simulink model "RoboBoatVU_2014_F"  (R2014a)
settings: Solver=FixedStepDiscrete  StartTime=0.0  StopTime=inf  FixedStep=.1  RelTol=1e-3
undefined symbols (not defined in the file): Com1, Com2, Com3, Com4, DiscIntNeverNeededParam, RGB24, standard
libraries: visiontextngfix x74, simulink x56, xpcseriallib x15, dspmtrx3 x14, slrtlib x3, speedgoatlib_IO102 x3, visionstatistics x2, dspstat3 x2, dspindex x2, xpcvideousblib x2, xpcvideoutillib x2, speedgoatlib x1
(part 7 of 7)

== system RoboBoatVU_2014_F/Main FSM/Start Speed Gate/Start Speed Gate Detection/Green Detection/Image Reduction ==
  HSV : Inport
  Cut Out Sky : dspmtrx3/Submatrix  RowSpan=Range of rows  RowStartMode=First  RowStartIndex=1  RowEndMode=Index  RowEndIndex=280  ColSpan=Range of columns  ColStartMode=First  ColStartIndex=1  ColEndMode=Last  ColEndIndex=1
  Cut Out Sky1 : dspmtrx3/Submatrix  RowSpan=Range of rows  RowStartMode=First  RowStartIndex=1  RowEndMode=Index  RowEndIndex=280  ColSpan=Range of columns  ColStartMode=First  ColStartIndex=1  ColEndMode=Last  ColEndIndex=1
  H : Selector  NumberOfDimensions=3  InputPortWidth=3  IndexOptions=Select all,Select all,Index vector (dialog)  Indices=[1 3],1,1  OutputSizes=1,1,1
  Logical Operator : Logic  AllPortsSameDT=off  OutDataTypeStr=boolean
  Logical Operator1 : Logic  AllPortsSameDT=off  OutDataTypeStr=boolean
  Logical Operator2 : Logic  AllPortsSameDT=off  OutDataTypeStr=boolean
  Upper limit : simulink/Logic and Bit Operations/Compare To Constant  relop=<=  const=110  OutDataTypeStr=boolean
  Upper limit1 : simulink/Logic and Bit Operations/Compare To Constant  relop=>=  const=90  OutDataTypeStr=boolean
  Upper limit2 : simulink/Logic and Bit Operations/Compare To Constant  relop=>=  const=60  OutDataTypeStr=boolean
  Upper limit3 : simulink/Logic and Bit Operations/Compare To Constant  relop=<=  const=160  OutDataTypeStr=boolean
  V : Selector  NumberOfDimensions=3  InputPortWidth=3  IndexOptions=Select all,Select all,Index vector (dialog)  Indices=[1 3],1,3  OutputSizes=1,1,1
  Green BW : Outport
  wires:
  H/1 -> Cut Out Sky/1
  HSV/1 -> V/1, H/1
  Cut Out Sky/1 -> Upper limit1/1, Upper limit/1
  Upper limit1/1 -> Logical Operator/2
  Upper limit/1 -> Logical Operator/1
  V/1 -> Cut Out Sky1/1
  Cut Out Sky1/1 -> Upper limit3/1, Upper limit2/1
  Logical Operator/1 -> Logical Operator1/1
  Logical Operator1/1 -> Green BW/1
  Upper limit2/1 -> Logical Operator2/1
  Upper limit3/1 -> Logical Operator2/2
  Logical Operator2/1 -> Logical Operator1/2

== system RoboBoatVU_2014_F/Main FSM/Start Speed Gate/Start Speed Gate Detection/Red Detection/Exclusions ==
  Area In : Inport
  Centroid In : Inport  Port=2
  BBox In : Inport  Port=3
  Extent In : Inport  Port=4
  Closest Blob : Subsystem
  Data Type Conversion : DataTypeConversion  OutDataTypeStr=double
  Extent Exclusion : Subsystem
  Height to Width Exclusion : Subsystem
  Logical Operator : Logic  AllPortsSameDT=off  OutDataTypeStr=boolean
  Variable Selector : dspindex/Variable Selector  NumInputs=3  rowsOrCols=Rows  IdxMode=Variable  Elements=[1 3]  ZerOneIdxMode=One-based  errmode=Clip Index  FillMode=on  FillValues=-1
  Centroid Out : Outport
  BBox Out : Outport  Port=2
  wires:
  Extent In/1 -> Extent Exclusion/1(Extent)
  BBox In/1 -> Data Type Conversion/1
  Height to Width Exclusion/1(Idx) -> Logical Operator/1
  Extent Exclusion/1(Idx) -> Logical Operator/2
  Logical Operator/1 -> Variable Selector/4
  Centroid In/1 -> Variable Selector/2
  Variable Selector/2 -> Closest Blob/2(Centroid In)
  Variable Selector/3 -> Closest Blob/3(BBox In)
  Closest Blob/1(Centroid Out) -> Centroid Out/1
  Closest Blob/2(BBox Out) -> BBox Out/1
  Data Type Conversion/1 -> Variable Selector/3, Height to Width Exclusion/1(BBox)
  Area In/1 -> Variable Selector/1
  Variable Selector/1 -> Closest Blob/1(Area In)

== system RoboBoatVU_2014_F/Main FSM/Start Speed Gate/Start Speed Gate Detection/Red Detection/Image Reduction ==
  HSV : Inport
  Cut Out Sky : dspmtrx3/Submatrix  RowSpan=Range of rows  RowStartMode=First  RowStartIndex=1  RowEndMode=Index  RowEndIndex=280  ColSpan=Range of columns  ColStartMode=First  ColStartIndex=1  ColEndMode=Last  ColEndIndex=1
  Cut Out Sky1 : dspmtrx3/Submatrix  RowSpan=Range of rows  RowStartMode=First  RowStartIndex=1  RowEndMode=Index  RowEndIndex=280  ColSpan=Range of columns  ColStartMode=First  ColStartIndex=1  ColEndMode=Last  ColEndIndex=1
  H : Selector  NumberOfDimensions=3  InputPortWidth=3  IndexOptions=Select all,Select all,Index vector (dialog)  Indices=[1 3],1,1  OutputSizes=1,1,1
  H Range 1 : simulink/Logic and Bit Operations/Compare To Constant  relop=<=  const=5  OutDataTypeStr=boolean
  H Range 2 : simulink/Logic and Bit Operations/Compare To Constant  relop=>=  const=0  OutDataTypeStr=boolean
  H Range 3 : simulink/Logic and Bit Operations/Compare To Constant  relop=<=  const=255  OutDataTypeStr=boolean
  H Range 4 : simulink/Logic and Bit Operations/Compare To Constant  relop=>=  const=220  OutDataTypeStr=boolean
  Logical Operator{,1,3..4} (4 alike) : Logic  AllPortsSameDT=off  OutDataTypeStr=boolean
  Logical Operator2 : Logic  Operator=OR  AllPortsSameDT=off  OutDataTypeStr=boolean
  V : Selector  NumberOfDimensions=3  InputPortWidth=3  IndexOptions=Select all,Select all,Index vector (dialog)  Indices=[1 3],1,3  OutputSizes=1,1,1
  V Range : simulink/Logic and Bit Operations/Compare To Constant  relop=>=  const=60  OutDataTypeStr=boolean
  V Range1 : simulink/Logic and Bit Operations/Compare To Constant  relop=<=  const=200  OutDataTypeStr=boolean
  Red BW : Outport
  wires:
  HSV/1 -> H/1, V/1
  H/1 -> Cut Out Sky/1
  Cut Out Sky/1 -> H Range 4/1, H Range 3/1, H Range 2/1, H Range 1/1
  V/1 -> Cut Out Sky1/1
  H Range 1/1 -> Logical Operator/1
  H Range 2/1 -> Logical Operator/2
  H Range 3/1 -> Logical Operator1/1
  H Range 4/1 -> Logical Operator1/2
  Logical Operator/1 -> Logical Operator2/1
  Logical Operator1/1 -> Logical Operator2/2
  Cut Out Sky1/1 -> V Range1/1, V Range/1
  Logical Operator2/1 -> Logical Operator3/1
  Logical Operator3/1 -> Red BW/1
  V Range/1 -> Logical Operator4/1
  V Range1/1 -> Logical Operator4/2
  Logical Operator4/1 -> Logical Operator3/2

== system RoboBoatVU_2014_F/Sinks/actuators/analog output/Subsystem/Heading Controller ==
  Heading Desired : Inport
  Compass Heading : Inport  Port=2
  Gain : Gain  Gain=-0.05
  MATLAB Function : MATLAB Function  TreatAsAtomicUnit=on
  Saturation : Saturate  UpperLimit=5  LowerLimit=0
  Sum : Sum  Inputs=++|
  Voltage Nuetral : Constant  Value=2.5
  Steering : Outport
  wires:
  Compass Heading/1 -> MATLAB Function/2(CompassHeading)
  Heading Desired/1 -> MATLAB Function/1(HeadingDesired)
  MATLAB Function/1(steering) -> Gain/1
  Gain/1 -> Sum/2
  Voltage Nuetral/1 -> Sum/1
  Sum/1 -> Saturation/1
  Saturation/1 -> Steering/1

== system RoboBoatVU_2014_F/Sinks/actuators/analog output/Subsystem/Propulsion Controller ==
  RPM : Inport
  Saturation : Saturate  UpperLimit=5  LowerLimit=0
  Sum : Sum  Inputs=++|
  Voltage Neutral : Constant  Value=2.5
  Volts / RPM : Gain  Gain=2.5/6000
  Propulsion : Outport
  wires:
  RPM/1 -> Volts / RPM/1
  Volts / RPM/1 -> Sum/2
  Voltage Neutral/1 -> Sum/1
  Sum/1 -> Saturation/1
  Saturation/1 -> Propulsion/1

== system RoboBoatVU_2014_F/Main FSM/Obstacle Navigation1/Obstacle Navigation/GPS: Bee Line/Approach/Output Heirarchy ==
  Nav Finished : Inport
  Desired Heading : Inport  Port=2
  Sensors : Inport  Port=3
  Annotated Image : Inport  Port=4
  Bus Creator : BusCreator  Inputs=3
  Bus Creator1 : BusCreator  Inputs=2
  Bus Creator2 : BusCreator  Inputs=3
  Bus Creator3 : BusCreator  Inputs=2
  Bus Creator4 : BusCreator  Inputs=2
  Due Sample Start : Constant  Value=0
  RPM Desired : Constant  Value=2000
  Ready to Read : Constant  Value=0
  Uno Power : Constant  Value=0
  Outputs : Outport
  wires:
  RPM Desired/1 -> Bus Creator/1  "RPM"
  Bus Creator/1 -> Bus Creator1/1  "Control Signals"
  Bus Creator2/1 -> Bus Creator/3  "Arduino Signals"
  Uno Power/1 -> Bus Creator2/2  "Uno Power"
  Desired Heading/1 -> Bus Creator/2  "Desired Heading"
  Bus Creator1/1 -> Bus Creator4/1  "Outputs"
  Annotated Image/1 -> Bus Creator1/2  "Annotated Image"
  Sensors/1 -> Bus Creator4/2  "Sensors"
  Bus Creator4/1 -> Bus Creator3/1  "Output Signals"
  Ready to Read/1 -> Bus Creator2/1  "Ready to Read"
  Due Sample Start/1 -> Bus Creator2/3  "Due Sample Start"
  Bus Creator3/1 -> Outputs/1
  Nav Finished/1 -> Bus Creator3/2  "Task Finished"

== system RoboBoatVU_2014_F/Main FSM/Obstacle Navigation1/Obstacle Navigation/GPS: Bee Line/Orient/Output Heirarchy1 ==
  Annotated Image : Inport
  Desired Heading : Inport  Port=2
  Sensors : Inport  Port=3
  Bus Creator : BusCreator  Inputs=3
  Bus Creator1 : BusCreator  Inputs=2
  Bus Creator2 : BusCreator  Inputs=3
  Bus Creator3 : BusCreator  Inputs=2
  Bus Creator4 : BusCreator  Inputs=2
  Due Sample Start : Constant  Value=0
  Finished : Constant  Value=0
  RPM Desired : Constant  Value=0
  Ready to Read : Constant  Value=0
  Uno Power : Constant  Value=0
  Outputs : Outport
  wires:
  RPM Desired/1 -> Bus Creator/1  "RPM"
  Bus Creator/1 -> Bus Creator1/1  "Control Signals"
  Bus Creator2/1 -> Bus Creator/3  "Arduino Signals"
  Uno Power/1 -> Bus Creator2/2  "Uno Power"
  Desired Heading/1 -> Bus Creator/2  "Desired Heading"
  Bus Creator1/1 -> Bus Creator4/1  "Outputs"
  Annotated Image/1 -> Bus Creator1/2  "Annotated Image"
  Sensors/1 -> Bus Creator4/2  "Sensors"
  Bus Creator4/1 -> Bus Creator3/1  "Output Signals"
  Ready to Read/1 -> Bus Creator2/1  "Ready to Read"
  Due Sample Start/1 -> Bus Creator2/3  "Due Sample Start"
  Bus Creator3/1 -> Outputs/1
  Finished/1 -> Bus Creator3/2  "Task Finished"

== system RoboBoatVU_2014_F/Main FSM/Start Speed Gate/Start Speed Gate Detection/Green Detection/Exclusions1/Closest Blob ==
  note: Sorts the list of viable buoys based on the Y location of the bounding box, those
      | with higher values are lower on the screen. The lower the blob is on the screen,
      | the closer it is to the boat, since all the buoys are floating on the surface of the water.
      | The submatrix then selects the centroid and bbox of the blob with the highest
      | Y value and passes it as the closest blob.
  Area In : Inport
  Centroid In : Inport  Port=2
  BBox In : Inport  Port=3
  BBox Select : dspmtrx3/Submatrix  RowSpan=One row  RowStartMode=First  RowStartIndex=1  RowEndMode=Last  RowEndIndex=1  ColSpan=Range of columns  ColStartMode=Index  ColStartIndex=3  ColEndMode=Last  ColEndIndex=1
  Centroid Select : dspmtrx3/Submatrix  RowSpan=One row  RowStartMode=First  RowStartIndex=1  RowEndMode=Last  RowEndIndex=1  ColSpan=Range of columns  ColStartMode=First  ColStartIndex=2  ColEndMode=Index  ColEndIndex=2
  Matrix Concatenate : Concatenate  Mode=Multidimensional array  ConcatenateDimension=2
  Permute Matrix : dspmtrx3/Permute Matrix  mode=Rows  ZeroOneIdxMode=One-based  errmode=Clip index  checkDims=off
  Sort : dspstat3/Sort  otype=Index  dir=Descending  sortAlg=Quick sort  accumDataTypeStr=Inherit: Same as product output  accumLastDataTypeStr=Inherit: Same as product output  roundingMode=Floor  overflowMode=off
  Centroid Out : Outport
  BBox Out : Outport  Port=2
  wires:
  Centroid In/1 -> Matrix Concatenate/1
  BBox In/1 -> Matrix Concatenate/2
  Matrix Concatenate/1 -> Permute Matrix/1
  Sort/1 -> Permute Matrix/2
  Permute Matrix/1 -> BBox Select/1, Centroid Select/1
  BBox Select/1 -> BBox Out/1
  Centroid Select/1 -> Centroid Out/1
  Area In/1 -> Sort/1

== system RoboBoatVU_2014_F/Main FSM/Start Speed Gate/Start Speed Gate Detection/Green Detection/Exclusions1/Extent Exclusion ==
  note: Pixels Occpied by blob within bounding box should
      | be within a certain ratio for buoy
  Extent : Inport
  Logical Operator : Logic  AllPortsSameDT=off  OutDataTypeStr=boolean
  Lower limit : simulink/Logic and Bit Operations/Compare To Constant  relop=>=  const=0.4  OutDataTypeStr=boolean
  Upper limit : simulink/Logic and Bit Operations/Compare To Constant  relop=<=  const=0.9  OutDataTypeStr=boolean
  Idx : Outport
  wires:
  Extent/1 -> Lower limit/1, Upper limit/1
  Upper limit/1 -> Logical Operator/1
  Lower limit/1 -> Logical Operator/2
  Logical Operator/1 -> Idx/1

== system RoboBoatVU_2014_F/Main FSM/Start Speed Gate/Start Speed Gate Detection/Green Detection/Exclusions1/Height to Width Exclusion ==
  note: Buoys can be percieved significantly taller than they are wide
      | due to relfections in the water, but should not be percieved
      | much wider than they are tall - even in oversaturated lighting
      | conditions (which generally cuts off some height, but doesn't
      | effect width)
  BBox : Inport
  Divide : Product  Inputs=*/
  Height : dspmtrx3/Submatrix  RowSpan=All rows  RowStartMode=First  RowStartIndex=1  RowEndMode=Last  RowEndIndex=1  ColSpan=One column  ColStartMode=Index  ColStartIndex=4  ColEndMode=Last  ColEndIndex=1
  Logical Operator : Logic  AllPortsSameDT=off  OutDataTypeStr=boolean
  Width : dspmtrx3/Submatrix  RowSpan=All rows  RowStartMode=First  RowStartIndex=1  RowEndMode=Last  RowEndIndex=1  ColSpan=One column  ColStartMode=Index  ColStartIndex=3  ColEndMode=Last  ColEndIndex=1
  ratio max : simulink/Logic and Bit Operations/Compare To Constant  relop=<=  const=5  OutDataTypeStr=boolean
  ratio min : simulink/Logic and Bit Operations/Compare To Constant  relop=>=  const=1.5  OutDataTypeStr=boolean
  Idx : Outport
  wires:
  BBox/1 -> Height/1, Width/1
  Height/1 -> Divide/1
  Width/1 -> Divide/2
  Divide/1 -> ratio min/1, ratio max/1
  ratio max/1 -> Logical Operator/1
  ratio min/1 -> Logical Operator/2
  Logical Operator/1 -> Idx/1

== system RoboBoatVU_2014_F/Main FSM/Start Speed Gate/Start Speed Gate Detection/Red Detection/Exclusions/Closest Blob ==
  note: Sorts the list of viable buoys based on the Y location of the bounding box, those
      | with higher values are lower on the screen. The lower the blob is on the screen,
      | the closer it is to the boat, since all the buoys are floating on the surface of the water.
      | The submatrix then selects the centroid and bbox of the blob with the highest
      | Y value and passes it as the closest blob.
  Area In : Inport
  Centroid In : Inport  Port=2
  BBox In : Inport  Port=3
  BBox Select : dspmtrx3/Submatrix  RowSpan=One row  RowStartMode=First  RowStartIndex=1  RowEndMode=Last  RowEndIndex=1  ColSpan=Range of columns  ColStartMode=Index  ColStartIndex=3  ColEndMode=Last  ColEndIndex=1
  Centroid Select : dspmtrx3/Submatrix  RowSpan=One row  RowStartMode=First  RowStartIndex=1  RowEndMode=Last  RowEndIndex=1  ColSpan=Range of columns  ColStartMode=First  ColStartIndex=2  ColEndMode=Index  ColEndIndex=2
  Matrix Concatenate : Concatenate  Mode=Multidimensional array  ConcatenateDimension=2
  Permute Matrix : dspmtrx3/Permute Matrix  mode=Rows  ZeroOneIdxMode=One-based  errmode=Clip index  checkDims=off
  Sort : dspstat3/Sort  otype=Index  dir=Descending  sortAlg=Quick sort  accumDataTypeStr=Inherit: Same as product output  accumLastDataTypeStr=Inherit: Same as product output  roundingMode=Floor  overflowMode=off
  Centroid Out : Outport
  BBox Out : Outport  Port=2
  wires:
  Centroid In/1 -> Matrix Concatenate/1
  BBox In/1 -> Matrix Concatenate/2
  Area In/1 -> Sort/1
  Matrix Concatenate/1 -> Permute Matrix/1
  Sort/1 -> Permute Matrix/2
  Permute Matrix/1 -> BBox Select/1, Centroid Select/1
  BBox Select/1 -> BBox Out/1
  Centroid Select/1 -> Centroid Out/1

== system RoboBoatVU_2014_F/Main FSM/Start Speed Gate/Start Speed Gate Detection/Red Detection/Exclusions/Extent Exclusion ==
  note: Pixels Occpied by blob within bounding box should
      | be within a certain ratio for buoy
  Extent : Inport
  Logical Operator : Logic  AllPortsSameDT=off  OutDataTypeStr=boolean
  Lower limit : simulink/Logic and Bit Operations/Compare To Constant  relop=>=  const=0.35  OutDataTypeStr=boolean
  Upper limit : simulink/Logic and Bit Operations/Compare To Constant  relop=<=  const=0.9  OutDataTypeStr=boolean
  Idx : Outport
  wires:
  Upper limit/1 -> Logical Operator/1
  Lower limit/1 -> Logical Operator/2
  Logical Operator/1 -> Idx/1
  Extent/1 -> Lower limit/1, Upper limit/1

== system RoboBoatVU_2014_F/Main FSM/Start Speed Gate/Start Speed Gate Detection/Red Detection/Exclusions/Height to Width Exclusion ==
  note: Buoys can be percieved significantly taller than they are wide
      | due to relfections in the water, but should not be percieved
      | much wider than they are tall - even in oversaturated lighting
      | conditions (which generally cuts off some height, but doesn't
      | effect width)
  BBox : Inport
  Divide : Product  Inputs=*/
  Height : dspmtrx3/Submatrix  RowSpan=All rows  RowStartMode=First  RowStartIndex=1  RowEndMode=Last  RowEndIndex=1  ColSpan=One column  ColStartMode=Index  ColStartIndex=4  ColEndMode=Last  ColEndIndex=1
  Logical Operator : Logic  AllPortsSameDT=off  OutDataTypeStr=boolean
  Width : dspmtrx3/Submatrix  RowSpan=All rows  RowStartMode=First  RowStartIndex=1  RowEndMode=Last  RowEndIndex=1  ColSpan=One column  ColStartMode=Index  ColStartIndex=3  ColEndMode=Last  ColEndIndex=1
  ratio max : simulink/Logic and Bit Operations/Compare To Constant  relop=<=  const=5  OutDataTypeStr=boolean
  ratio min : simulink/Logic and Bit Operations/Compare To Constant  relop=>=  const=1.5  OutDataTypeStr=boolean
  Idx : Outport
  wires:
  BBox/1 -> Height/1, Width/1
  Height/1 -> Divide/1
  Width/1 -> Divide/2
  Divide/1 -> ratio min/1, ratio max/1
  ratio max/1 -> Logical Operator/1
  ratio min/1 -> Logical Operator/2
  Logical Operator/1 -> Idx/1

== matlab function RoboBoatVU_2014_F/Main FSM/Main Enabler ==
  data: taskSelector output; initEn output; commEn output; colorSeqEn output; ssGateEn output; obstNavEn output; acouLocEn output; dockEn output; rtnEn output; RCEn output; mainTask input; RCHold input; initFin input; commFin input; colorSeqFin input; ssGateFin input; obstNavFin input; acouLocFin input; dockFin input; rtnFin input; termEn output
function [taskSelector,initEn,commEn,colorSeqEn,ssGateEn,obstNavEn,...
    acouLocEn,dockEn,rtnEn,RCEn,termEn] = taskEnabler(mainTask,RCHold,initFin,...
    commFin,colorSeqFin,ssGateFin,obstNavFin,acouLocFin,dockFin,rtnFin)
%Written by Anderson Lebbad on July 19, 2013
%Last Edited: Edward Zhu on June 2, 2014
%   Substring search for task was written in
%   Case switches were redundant, combined with first set of if statements

%Changes the value of MainMode and the enablers for the tasks within the
%Main FSM.

% Initialize enable signals
RCEn = 0;
initEn = 0;
commEn = 0;
colorSeqEn = 0;
ssGateEn = 0;
obstNavEn = 0;
acouLocEn = 0;
dockEn = 0;
rtnEn = 0;
termEn = 0;

% Convert main task indicator to a string
mainTaskStr = char(mainTask);

% Adjust finished states based on user task selection
if ~isempty(strfind(mainTaskStr,'Comm'))
    initFin = 1;
elseif ~isempty(strfind(mainTaskStr,'Color'))
    initFin = 1;
    commFin = 1;
elseif ~isempty(strfind(mainTaskStr,'SSGate'))
    initFin = 1;
    commFin = 1;
    colorSeqFin = 1;
elseif ~isempty(strfind(mainTaskStr,'Obstacle'))
    initFin = 1;
    commFin = 1;
    colorSeqFin = 1;
    ssGateFin = 1;
elseif ~isempty(strfind(mainTaskStr,'Acoustic'))
    initFin = 1;
    commFin = 1;
    colorSeqFin = 1;
    ssGateFin = 1;
    obstNavFin = 1;
elseif ~isempty(strfind(mainTaskStr,'Dock'))
    initFin = 1;
    commFin = 1;
    colorSeqFin = 1;
    ssGateFin = 1;
    obstNavFin = 1;
    acouLocFin = 1;
elseif ~isempty(strfind(mainTaskStr,'Return'))
    initFin = 1;
    commFin = 1;
    colorSeqFin = 1;
    ssGateFin = 1;
    obstNavFin = 1;
    acouLocFin = 1;
    dockFin = 1;
end

% Set enable signals based on state completion
if initFin == 0
    initEn = 1;
    taskSelector = 1;
elseif RCHold == 0
    RCEn = 1;
    taskSelector = 9;
elseif commFin == 0
    commEn = 1;
    taskSelector = 2;
elseif colorSeqFin == 0
    colorSeqEn = 1;
    taskSelector = 3;
elseif ssGateFin == 0
    ssGateEn = 1;
    taskSelector = 4;
elseif obstNavFin == 0
    obstNavEn = 1;
    taskSelector = 5;
elseif acouLocFin == 0
    acouLocEn = 1;
    taskSelector = 6;
elseif dockFin == 0
    dockEn = 1;
    taskSelector = 7;
elseif rtnFin == 0
    rtnEn = 1;
    taskSelector = 8;
else
    termEn = 1;
    taskSelector = 10;
end

== matlab function RoboBoatVU_2014_F/Main FSM/Start Speed Gate/Start Speed Gate Detection/Green Detection/y-shift ==
  data: CentroidIn input; CentroidOut output; BBoxIn input; BBoxOut output
function [CentroidOut, BBoxOut] = yShift(CentroidIn, BBoxIn)

%Written by Anderson Lebbad on July 24, 2013
%Last Edited: Anderson Lebbad on August 4, 2013
%   Renamed the function to match other instances

%This function compensates for the amount of the image that was cut out
%when the sky was removed by the image reduction subsystem

CentroidOut = [CentroidIn(1), CentroidIn(2)+175];
BBoxOut = [BBoxIn(1), BBoxIn(2)+175, BBoxIn(3:4)];

== matlab function RoboBoatVU_2014_F/Sinks/actuators/analog output/Subsystem/Heading Controller/MATLAB Function ==
  data: HeadingDesired input; steering output; CompassHeading input
function steering = CalcSteering(HeadingDesired, CompassHeading)

%Written by Anderson Lebbad on July 19, 2013
%Last Edited: Anderson Lebbad on August 14, 2013
%   Simplified using mod division

%Calculates the difference between the desired and current heading to be
%used for steering


%difference is calculated in the range of -180 to 180
steering = mod(HeadingDesired - CompassHeading, 360);
if steering > 180
    steering = steering - 360;
end

== matlab function RoboBoatVU_2014_F/Main FSM/Start Speed Gate/Start Speed Gate Detection/Red Detection/y-shift ==
  data: CentroidIn input; CentroidOut output; BBoxIn input; BBoxOut output
function [CentroidOut, BBoxOut] = yShift(CentroidIn, BBoxIn)

%Written by Anderson Lebbad on July 24, 2013
%Last Edited: Anderson Lebbad on August 4, 2013
%   Renamed the function to match other instances

%This function compensates for the amount of the image that was cut out
%when the sky was removed by the image reduction subsystem

CentroidOut = [CentroidIn(1), CentroidIn(2)+175];
BBoxOut = [BBoxIn(1), BBoxIn(2)+175, BBoxIn(3:4)];

== matlab function RoboBoatVU_2014_F/Main FSM/Obstacle Navigation1/Exit Gate/Gate 1 (Red & White)/Distance ==
  data: Distance output; DesiredGPS input; GPSLat input; GPSLong input
function Distance  = DistCalc(DesiredGPS, GPSLat, GPSLong)

%Written by Anderson Lebbad on July 22, 2013
%Last Edited:

%Orients the boat towards a target GPS point before approaching it.
%This is done to keep the approach angle minimal, so the approach
%algorithm does not circle the target and never reach it.

%Parse input GPS and convert angles to radians
CurLat = (floor(GPSLat/100)+mod(GPSLat,100)/60)*pi/180;
CurLong = (floor(GPSLong/100)+mod(GPSLong,100)/60)*pi/180;
DesLat = (floor(DesiredGPS(1)/100)+mod(DesiredGPS(1),100)/60)*pi/180;
DesLong = (floor(DesiredGPS(2)/100)+mod(DesiredGPS(2),100)/60)*pi/180;
%Difference between lats and longs
DiffLat = DesLat - CurLat;
MidLat = cos((CurLat + DesLat)/2);
DiffLong = DesLong - CurLong;
%Radius of the earth in meters
R = 6378137;

%Calculate distance using the great-circle distance formula
%Formula documented here:
%   http://www.movable-type.co.uk/scripts/latlong.html
% a = sin(DiffLat/2)^2+sin(DiffLong/2)^2*cos(CurLat)*cos(DesLat);
% c = 2*atan2(sqrt(a), sqrt(1-a));
% Distance = R*c;

%Calculating distance using Pythagora's
a = DiffLong*MidLat;
b = DiffLat;
Distance = R*sqrt(a^2+b^2);

== matlab function RoboBoatVU_2014_F/Main FSM/Obstacle Navigation1/Exit Gate/Gate 1 (Red & White)/MATLAB Function ==
  data: Prob input; RPM output; ColorID input; Dist input; Ang input; CurrentHeading input; GPSLat input; GPSLong input; Timer input; DesiredHeading output; gateGPS output
function [RPM,DesiredHeading,gateGPS] = navigation(Prob,ColorID,Dist,Ang,CurrentHeading,GPSLat,GPSLong,Timer)

% Function performs one buoy navigation through the start speed gates. If
% no buoys are found by the LIDAR/Vision assembly then an incremented
% turning algorithm is executed to turn by 10 degrees per increment up to 
% 90 degrees either way of the inital heading

% Written by Edward Zhu

persistent LockHeading TimeLastFound Counter Turn TurnInc gateLat gateLong

if isempty(LockHeading) && isempty(TimeLastFound) && isempty(Counter) && isempty(Turn) && isempty(TurnInc)
    LockHeading = CurrentHeading;
    TimeLastFound = 0;
    Counter = 0;
    TurnInc = 30;
    Turn = TurnInc;
    gateLat = 0;
    gateLong = 0;
end

Distance = Dist/100;

BoatWidth = 0.75;
Buffer = atan(2*BoatWidth/Distance);

RedOffset = Ang + Buffer;
WhiteOffset = Ang - Buffer;

R = 6378137;

CurLat = (floor(GPSLat/100)+mod(GPSLat,100)/60)*pi/180;
CurLong = (ceil(GPSLong/100)-mod(-GPSLong,100)/60)*pi/180;

gateHeading = (mod(CurrentHeading + Ang, 360))*pi/180;

if ColorID == 1 && Prob > 0.9
    if Ang < 0
        DesiredHeading = mod(CurrentHeading - RedOffset, 360);
    else
        DesiredHeading = mod(CurrentHeading + RedOffset, 360);
    end
    RPM = 4000;
    GateFound = 1;
    TimeLastFound = Timer;
    gateLat =  asin(sin(CurLat)*cos(Distance/R) + cos(CurLat)*sin(Distance/R)*cos(gateHeading))*180/pi;
    gateLong = (CurLong + atan2(sin(gateHeading)*sin(Distance/R)*cos(CurLat),cos(Distance/R)-sin(CurLat)*sin(gateLat)))*180/pi;
elseif ColorID == 2 && Prob > 0.9
    DesiredHeading = mod(LockHeading - Turn, 360);
    RPM = 0;
    GateFound = 1;
    TimeLastFound = Timer;
%     DesiredHeading = mod(CurrentHeading - WhiteOffset, 360);
%     RPM = 4000;
%     GateFound = 1;
%     TimeLastFound = Timer;
%     gateLat =  asin(sin(CurLat)*cos(Distance/R) + cos(CurLat)*sin(Distance/R)*cos(gateHeading))*180/pi;
%     gateLong = (CurLong + atan2(sin(gateHeading)*sin(Distance/R)*cos(CurLat),cos(Distance/R)-sin(CurLat)*sin(gateLat)))*180/pi;
else
    DesiredHeading = CurrentHeading;
    RPM = 0;
    GateFound = 0;
end

gateGPS = [gateLat gateLong];
TimeNoBuoys = Timer - TimeLastFound;

if GateFound == 0 && TimeNoBuoys > 15
    RPM = 0;
    DesiredHeading = mod(LockHeading - Turn, 360);
    HeadingDiff = DesiredHeading - CurrentHeading;
    gateGPS = [gateLat gateLong];
    
    if HeadingDiff > 180
        HeadingDiff = HeadingDiff - 360;
    elseif HeadingDiff < -180
        HeadingDiff = HeadingDiff + 360;
    end
    
    if HeadingDiff < 3
        Counter = Counter + 1;
    else
        Counter = 0;
    end
    
    if Counter >= 15
        Turn = Turn + TurnInc;
        Counter = 0;
        if abs(Turn) > 90
            TurnInc = -TurnInc;
        end
    end
end

== matlab function RoboBoatVU_2014_F/Main FSM/Obstacle Navigation1/Exit Gate/Gate 3 (White & Green)/MATLAB Function ==
  data: Prob input; RPM output; ColorID input; Dist input; Ang input; CurrentHeading input; GPSLat input; GPSLong input; Timer input; DesiredHeading output; gateGPS output
function [RPM,DesiredHeading,gateGPS] = navigation(Prob,ColorID,Dist,Ang,CurrentHeading,GPSLat,GPSLong,Timer)

% Function performs one buoy navigation through the start speed gates. If
% no buoys are found by the LIDAR/Vision assembly then an incremented
% turning algorithm is executed to turn by 10 degrees per increment up to 
% 90 degrees either way of the inital heading

% Written by Edward Zhu


persistent LockHeading TimeLastFound Counter Turn TurnInc gateLat gateLong

if isempty(LockHeading) && isempty(TimeLastFound) && isempty(Counter) && isempty(Turn) && isempty(TurnInc)
    LockHeading = CurrentHeading;
    TimeLastFound = 0;
    Counter = 0;
    TurnInc = 30;
    Turn = TurnInc;
    gateLat = 0;
    gateLong = 0;
end
Distance = Dist/100;
BoatWidth = 0.75;
Buffer = atan(2*BoatWidth/Distance);

WhiteOffset = Ang + Buffer;
GreenOffset = Ang - Buffer;

R = 6378137;

CurLat = (floor(GPSLat/100)+mod(GPSLat,100)/60)*pi/180;
CurLong = (ceil(GPSLong/100)-mod(-GPSLong,100)/60)*pi/180;

gateHeading = (mod(CurrentHeading - Ang, 360))*pi/180;

if ColorID == 2 && Prob > 0.9
    DesiredHeading = mod(LockHeading - Turn, 360);
    RPM = 0;
    GateFound = 1;
    TimeLastFound = Timer;
elseif ColorID == 3 && Prob > 0.9
    if Ang > 0
        DesiredHeading = mod(CurrentHeading - GreenOffset, 360);
    else
        DesiredHeading = mod(CurrentHeading + GreenOffset, 360);
    end
    RPM = 4000;
    GateFound = 1;
    TimeLastFound = Timer;
    gateLat =  asin(sin(CurLat)*cos(Distance/R) + cos(CurLat)*sin(Distance/R)*cos(gateHeading))*180/pi;
    gateLong = (CurLong + atan2(sin(gateHeading)*sin(Distance/R)*cos(CurLat),cos(Distance/R)-sin(CurLat)*sin(gateLat)))*180/pi;
else
    DesiredHeading = CurrentHeading;
    RPM = 0;
    GateFound = 0;
end

gateGPS = [gateLat gateLong];
TimeNoBuoys = Timer - TimeLastFound;

if GateFound == 0 && TimeNoBuoys > 15
    RPM = 0;
    DesiredHeading = mod(LockHeading - Turn, 360);
    HeadingDiff = DesiredHeading - CurrentHeading;
    gateGPS = [gateLat gateLong];
    
    if HeadingDiff > 180
        HeadingDiff = HeadingDiff - 360;
    elseif HeadingDiff < -180
        HeadingDiff = HeadingDiff + 360;
    end
    
    if HeadingDiff < 3
        Counter = Counter + 1;
    else
        Counter = 0;
    end
    
    if Counter >= 15
        Turn = Turn + TurnInc;
        Counter = 0;
        if abs(Turn) > 90
            TurnInc = -TurnInc;
        end
    end
end

== matlab function RoboBoatVU_2014_F/Main FSM/Obstacle Navigation1/Enter Gate/Gate 1 (Red & White)/MATLAB Function ==
  data: Prob input; RPM output; ColorID input; Dist input; Ang input; CurrentHeading input; GPSLat input; GPSLong input; Timer input; DesiredHeading output; gateGPS output
function [RPM,DesiredHeading,gateGPS] = navigation(Prob,ColorID,Dist,Ang,CurrentHeading,GPSLat,GPSLong,Timer)

% Function performs one buoy navigation through the start speed gates. If
% no buoys are found by the LIDAR/Vision assembly then an incremented
% turning algorithm is executed to turn by 10 degrees per increment up to 
% 90 degrees either way of the inital heading

% Written by Edward Zhu

persistent LockHeading TimeLastFound Counter Turn TurnInc gateLat gateLong

if isempty(LockHeading) && isempty(TimeLastFound) && isempty(Counter) && isempty(Turn) && isempty(TurnInc)
    LockHeading = CurrentHeading;
    TimeLastFound = 0;
    Counter = 0;
    TurnInc = 30;
    Turn = TurnInc;
    gateLat = 0;
    gateLong = 0;
end

Distance = Dist/100;

BoatWidth = 0.75;
Buffer = atan(2*BoatWidth/Distance);

RedOffset = Ang + Buffer;
WhiteOffset = Ang - Buffer;

R = 6378137;

CurLat = (floor(GPSLat/100)+mod(GPSLat,100)/60)*pi/180;
CurLong = (ceil(GPSLong/100)-mod(-GPSLong,100)/60)*pi/180;

gateHeading = (mod(CurrentHeading + Ang, 360))*pi/180;

if ColorID == 1 && Prob > 0.9
    if Ang < 0
        DesiredHeading = mod(CurrentHeading - RedOffset, 360);
    else
        DesiredHeading = mod(CurrentHeading + RedOffset, 360);
    end
    RPM = 4000;
    GateFound = 1;
    TimeLastFound = Timer;
    gateLat =  asin(sin(CurLat)*cos(Distance/R) + cos(CurLat)*sin(Distance/R)*cos(gateHeading))*180/pi;
    gateLong = (CurLong + atan2(sin(gateHeading)*sin(Distance/R)*cos(CurLat),cos(Distance/R)-sin(CurLat)*sin(gateLat)))*180/pi;
elseif ColorID == 2 && Prob > 0.9
    DesiredHeading = mod(LockHeading - Turn, 360);
    RPM = 0;
    GateFound = 1;
    TimeLastFound = Timer;
%     DesiredHeading = mod(CurrentHeading - WhiteOffset, 360);
%     RPM = 4000;
%     GateFound = 1;
%     TimeLastFound = Timer;
%     gateLat =  asin(sin(CurLat)*cos(Distance/R) + cos(CurLat)*sin(Distance/R)*cos(gateHeading))*180/pi;
%     gateLong = (CurLong + atan2(sin(gateHeading)*sin(Distance/R)*cos(CurLat),cos(Distance/R)-sin(CurLat)*sin(gateLat)))*180/pi;
else
    DesiredHeading = CurrentHeading;
    RPM = 0;
    GateFound = 0;
end

gateGPS = [gateLat gateLong];
TimeNoBuoys = Timer - TimeLastFound;

if GateFound == 0 && TimeNoBuoys > 15
    RPM = 0;
    DesiredHeading = mod(LockHeading - Turn, 360);
    HeadingDiff = DesiredHeading - CurrentHeading;
    gateGPS = [gateLat gateLong];
    
    if HeadingDiff > 180
        HeadingDiff = HeadingDiff - 360;
    elseif HeadingDiff < -180
        HeadingDiff = HeadingDiff + 360;
    end
    
    if HeadingDiff < 3
        Counter = Counter + 1;
    else
        Counter = 0;
    end
    
    if Counter >= 15
        Turn = Turn + TurnInc;
        Counter = 0;
        if abs(Turn) > 90
            TurnInc = -TurnInc;
        end
    end
end

== matlab function RoboBoatVU_2014_F/Main FSM/Communication/Docking Bay Comm/MATLAB Function ==
  data: requestNumOut output; CP input; requestNumIn input; Finished output
function [requestNumOut, Finished] = requestSender(CP, requestNumIn)

if CP < 1
    requestNumOut = requestNumIn;
    Finished = 0;
else
    requestNumOut = 0;
    Finished = 1;
end
end

== matlab function RoboBoatVU_2014_F/Main FSM/Obstacle Navigation2/MATLAB Function ==
  data: requestNumOut output; CP input; requestNumIn input; Finished output
function [requestNumOut, Finished] = requestSender(CP, requestNumIn)

persistent counter
if isempty(counter)
    counter = 0;
end

if CP < 1
    requestNumOut = requestNumIn;
    Finished = 0;
else
    counter = counter + 1;
    if counter >= 50
        requestNumOut = 0;
        Finished = 1;
    else
        requestNumOut = requestNumIn;
        Finished = 0;
    end
end

== matlab function RoboBoatVU_2014_F/Main FSM/Obstacle Navigation1/GPS: Center/Orient/Within Range ==
  data: DesiredHeading input; Finished output; Compass input
function Finished = OrientLocked(DesiredHeading, Compass)

%Written by Anderson Lebbad on July 22, 2013
%Last Edited:

%This function checks to see if the target heading has been reached and 
%sends a finished signal when it has.

HeadingDiff = DesiredHeading - Compass;

%Sets the range for the difference angle to be -180 to +180
if HeadingDiff > 180
    HeadingDiff = HeadingDiff - 360;
elseif HeadingDiff < -180
    HeadingDiff = HeadingDiff + 360;
end

%If the Heading is within 3 degrees, the angle is close enough to send a
%finished signal
if abs(HeadingDiff) < 3
    Finished = 1;
else
    Finished = 0;
end

== matlab function RoboBoatVU_2014_F/Main FSM/Obstacle Navigation1/Obstacle Navigation/GPS: Bee Line/Approach/Desired Heading and Distance ==
  data: Distance output; DesiredGPS input; DesiredHeading output; GPSLat input; GPSLong input
function [Distance, DesiredHeading] = Approach(DesiredGPS, GPSLat, GPSLong)

%Written by Anderson Lebbad on July 22, 2013
%Last Edited: Edward Zhu July 5, 2014

%Edit:
% Switched from great-circle distance formula to equirectangular approx and
%used mod for desired heading
% Changed calculation to use positve lat and negative long

%Orients the boat towards a target GPS point before approaching it.
%This is done to keep the approach angle minimal, so the approach
%algorithm does not circle the target and never reach it.

%Parse input GPS and convert angles to radians
CurLat = (floor(GPSLat/100)+mod(GPSLat,100)/60)*pi/180;
CurLong = (ceil(GPSLong/100)-mod(-GPSLong,100)/60)*pi/180;
DesLat = (floor(DesiredGPS(1)/100)+mod(DesiredGPS(1),100)/60)*pi/180;
DesLong = (ceil(DesiredGPS(2)/100)-mod(-DesiredGPS(2),100)/60)*pi/180;

%Difference between lats and longs
DiffLat = DesLat - CurLat;
MidLat = cos((CurLat + DesLat)/2);
DiffLong = DesLong - CurLong;

%Radius of the earth in meters
R = 6378137;

%Calculate distance using the great-circle distance formula
%Formula documented here:
%   http://www.movable-type.co.uk/scripts/latlong.html
% a = sin(DiffLat/2)^2+sin(DiffLong/2)^2*cos(CurLat)*cos(DesLat);
% c = 2*atan2(sqrt(a), sqrt(1-a));
% Distance = R*c;

%Calculating distance using equirectangular approximation since distances
%concerned are very small
a = DiffLong*MidLat;
b = DiffLat;
Distance = R*sqrt(a^2+b^2);

%Calculate initial bearing - formula documented here: 
%   http://www.movable-type.co.uk/scripts/latlong.html
y = sin(DiffLong)*cos(DesLat);
x = cos(CurLat)*sin(DesLat)-sin(CurLat)*cos(DesLat)*cos(DiffLong);
DesiredHeading = mod(atan2(y, x)*180/pi + 360, 360);

== matlab function RoboBoatVU_2014_F/Main FSM/Acoustic Location1/GPS: Acoustic Center1/Orient/Within Range ==
  data: DesiredHeading input; Finished output; Compass input
function Finished = OrientLocked(DesiredHeading, Compass)

%Written by Anderson Lebbad on July 22, 2013
%Last Edited:

%This function checks to see if the target heading has been reached and 
%sends a finished signal when it has.
persistent counter
if isempty(counter)
    counter = 0;
end

HeadingDiff = DesiredHeading - Compass;

%Sets the range for the difference angle to be -180 to +180
if HeadingDiff > 180
    HeadingDiff = HeadingDiff - 360;
elseif HeadingDiff < -180
    HeadingDiff = HeadingDiff + 360;
end

%If the Heading is within 3 degrees, the angle is close enough to send a
%finished signal
if abs(HeadingDiff) < 4
    counter = counter + 1;
    if counter >= 10;
        Finished = 1;
    else
        Finished = 0;
    end
else
    counter = 0;
    Finished = 0;
end

== matlab function RoboBoatVU_2014_F/Main FSM/Docking/GPS: Acoustic Center1/GPS Enabler ==
  data: Finished input; GPSMode output; OrientEn output; ApproachEn output
function [GPSMode, OrientEn, ApproachEn] = GPSEnable(Finished)

%Written by Anderson Lebbad on July 22, 2013
%Last Edited: July 27, 2013
%   Removed Termination Block

%This function enables GPS tasks. First the boat orients towards the
%target, then it approaches it.


%Parse Finished signal
OrientFinished = Finished(1);


%Initialize Enablers
OrientEn = 0;
ApproachEn = 0;


%Switches the enable signal based on which task is flagged as done.
if OrientFinished == 0
    OrientEn = 1;
    GPSMode = 1;
else
    ApproachEn = 1;
    GPSMode = 2;
end

== matlab function RoboBoatVU_2014_F/Main FSM/Acoustic Location1/GPS: Acoustic Center1/Approach/Desired Heading and Distance ==
  data: Distance output; DesiredGPS input; DesiredHeading output; GPSLat input; GPSLong input
function [Distance, DesiredHeading] = Approach(DesiredGPS, GPSLat, GPSLong)

%Written by Anderson Lebbad on July 22, 2013
%Last Edited: Edward Zhu July 5, 2014

%Edit:
% Switched from great-circle distance formula to equirectangular approx and
%used mod for desired heading
% Changed calculation to use positve lat and negative long

%Orients the boat towards a target GPS point before approaching it.
%This is done to keep the approach angle minimal, so the approach
%algorithm does not circle the target and never reach it.

%Parse input GPS and convert angles to radians
CurLat = (floor(GPSLat/100)+mod(GPSLat,100)/60)*pi/180;
CurLong = (ceil(GPSLong/100)-mod(-GPSLong,100)/60)*pi/180;
DesLat = (floor(DesiredGPS(1)/100)+mod(DesiredGPS(1),100)/60)*pi/180;
DesLong = (ceil(DesiredGPS(2)/100)-mod(-DesiredGPS(2),100)/60)*pi/180;

%Difference between lats and longs
DiffLat = DesLat - CurLat;
MidLat = cos((CurLat + DesLat)/2);
DiffLong = DesLong - CurLong;

%Radius of the earth in meters
R = 6378137;

%Calculate distance using the great-circle distance formula
%Formula documented here:
%   http://www.movable-type.co.uk/scripts/latlong.html
% a = sin(DiffLat/2)^2+sin(DiffLong/2)^2*cos(CurLat)*cos(DesLat);
% c = 2*atan2(sqrt(a), sqrt(1-a));
% Distance = R*c;

%Calculating distance using equirectangular approximation since distances
%concerned are very small
a = DiffLong*MidLat;
b = DiffLat;
Distance = R*sqrt(a^2+b^2);

%Calculate initial bearing - formula documented here: 
%   http://www.movable-type.co.uk/scripts/latlong.html
y = sin(DiffLong)*cos(DesLat);
x = cos(CurLat)*sin(DesLat)-sin(CurLat)*cos(DesLat)*cos(DiffLong);
DesiredHeading = mod(atan2(y, x)*180/pi + 360, 360);

== matlab function RoboBoatVU_2014_F/Main FSM/Acoustic Location1/GPS:Waypoint/Approach/Desired Heading and Distance ==
  data: Distance output; DesiredGPS input; DesiredHeading output; GPSLat input; GPSLong input
function [Distance, DesiredHeading] = Approach(DesiredGPS, GPSLat, GPSLong)

%Written by Anderson Lebbad on July 22, 2013
%Last Edited: Edward Zhu July 5, 2014

%Edit:
% Switched from great-circle distance formula to equirectangular approx and
%used mod for desired heading
% Changed calculation to use positve lat and negative long

%Orients the boat towards a target GPS point before approaching it.
%This is done to keep the approach angle minimal, so the approach
%algorithm does not circle the target and never reach it.

%Parse input GPS and convert angles to radians
CurLat = (floor(GPSLat/100)+mod(GPSLat,100)/60)*pi/180;
CurLong = (ceil(GPSLong/100)-mod(-GPSLong,100)/60)*pi/180;
DesLat = (floor(DesiredGPS(1)/100)+mod(DesiredGPS(1),100)/60)*pi/180;
DesLong = (ceil(DesiredGPS(2)/100)-mod(-DesiredGPS(2),100)/60)*pi/180;

%Difference between lats and longs
DiffLat = DesLat - CurLat;
MidLat = cos((CurLat + DesLat)/2);
DiffLong = DesLong - CurLong;

%Radius of the earth in meters
R = 6378137;

%Calculate distance using the great-circle distance formula
%Formula documented here:
%   http://www.movable-type.co.uk/scripts/latlong.html
% a = sin(DiffLat/2)^2+sin(DiffLong/2)^2*cos(CurLat)*cos(DesLat);
% c = 2*atan2(sqrt(a), sqrt(1-a));
% Distance = R*c;

%Calculating distance using equirectangular approximation since distances
%concerned are very small
a = DiffLong*MidLat;
b = DiffLat;
Distance = R*sqrt(a^2+b^2);

%Calculate initial bearing - formula documented here: 
%   http://www.movable-type.co.uk/scripts/latlong.html
y = sin(DiffLong)*cos(DesLat);
x = cos(CurLat)*sin(DesLat)-sin(CurLat)*cos(DesLat)*cos(DiffLong);
DesiredHeading = mod(atan2(y, x)*180/pi + 360, 360);

== matlab function RoboBoatVU_2014_F/Main FSM/Acoustic Location1/Task Option/Message Composer ==
  data: taskStrInit input; taskStrAdj output
function taskStrAdj = composeMessage(taskStrInit)
%Written by Anderson Lebbad on August 9, 2013
%Last Edited: Edward Zhu on June 2, 2014

%This function adjusts the length of a vector to a set value by filling
%the remaining space with 0's. This is necessary for data store objects
%that have a fixed size for the memory allocation, but a variable length
%input.

%Length of message packet
strLength = 8;

%Size of text in message
taskStrLength = size(taskStrInit,1);

%Pad end of text with zeros
taskStrAdj = [taskStrInit' zeros(1,strLength-taskStrLength)];

== matlab function RoboBoatVU_2014_F/Main FSM/Docking/GPS:Waypoint/Orient/Within Range ==
  data: DesiredHeading input; Finished output; Compass input
function Finished = OrientLocked(DesiredHeading, Compass)

%Written by Anderson Lebbad on July 22, 2013
%Last Edited:

%This function checks to see if the target heading has been reached and 
%sends a finished signal when it has.
persistent counter
if isempty(counter)
    counter = 0;
end

HeadingDiff = DesiredHeading - Compass;

%Sets the range for the difference angle to be -180 to +180
if HeadingDiff > 180
    HeadingDiff = HeadingDiff - 360;
elseif HeadingDiff < -180
    HeadingDiff = HeadingDiff + 360;
end

%If the Heading is within 3 degrees, the angle is close enough to send a
%finished signal
if abs(HeadingDiff) < 4
    counter = counter + 1;
    if counter >= 10;
        Finished = 1;
    else
        Finished = 0;
    end
else
    counter = 0;
    Finished = 0;
end
